simulink model "araba"  (R2020a)
settings: Solver=VariableStepAuto  StartTime=0.0  StopTime=10.0  RelTol=1e-3
settings Model: Creator=muham  LastModifiedBy=muham

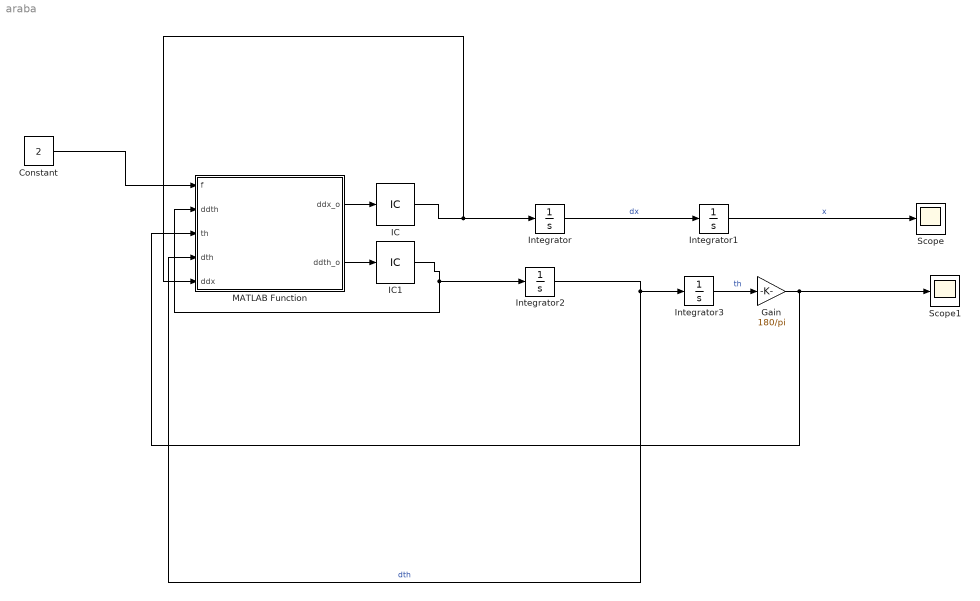
== system araba ==
  Constant : Constant  Value=2
  Gain : Gain  Gain=180/pi
  IC : InitialCondition  Value=0.0001
  IC1 : InitialCondition  Value=0.00001
  Integrator : Integrator  InitialCondition=5
  Integrator1 : Integrator
  Integrator2 : Integrator  InitialCondition=pi/3
  Integrator3 : Integrator
  MATLAB Function : MATLAB Function  TreatAsAtomicUnit=on
  Scope : Scope
  Scope1 : Scope
  wires:
  Integrator/1 -> Integrator1/1  "dx"
  MATLAB Function/1(ddx_o) -> IC/1
  MATLAB Function/2(ddth_o) -> IC1/1
  Integrator2/1 -> MATLAB Function/4(dth), Integrator3/1  "dth"
  Constant/1 -> MATLAB Function/1(f)
  Integrator3/1 -> Gain/1  "th"
  Integrator1/1 -> Scope/1  "x"
  IC/1 -> MATLAB Function/5(ddx), Integrator/1
  IC1/1 -> MATLAB Function/2(ddth), Integrator2/1
  Gain/1 -> MATLAB Function/3(th), Scope1/1

== matlab function araba/MATLAB Function ==
  data: f input; ddx_o output; ddth input; th input; dth input; ddx input; ddth_o output
function  [ddx_o,ddth_o] = oto_arc(f,ddth,th,dth,ddx)
f=2;
kp=0.35;
kc=2;
g=9.81;
l=0.75;

ddx_o=(f-kp*l*ddth*cos(th)+kp*l*dth.^2*sin(th))/(kp+kc)
ddth_o=(-kp*g*l*sin(th)-kp*l*ddx*cos(th))/(kp*l.^2)
end
